simulink model "scenario1_TAC_5robots_plus"  (R2020b)
settings: Solver=FixedStepAuto  StartTime=0.0  StopTime=40.0  FixedStep=1e-2  RelTol=1e-3
libraries: simulink x6
(part 1 of 2)
settings Model: Creator=Admin  LastModifiedBy=Admin

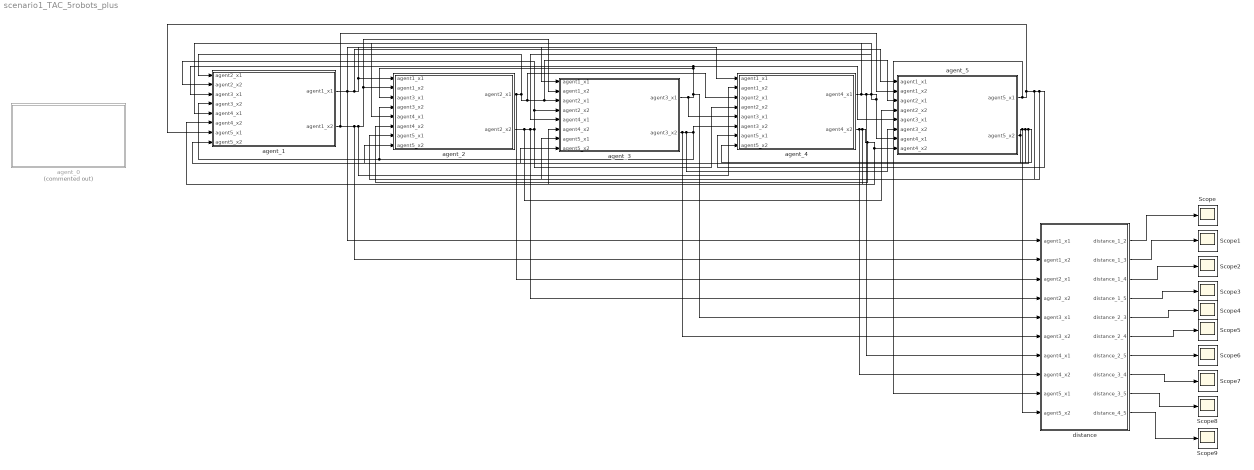
== system scenario1_TAC_5robots_plus ==
  Scope{,1..9} (10 alike) : Scope
  agent_0 : Subsystem  Commented=on
  agent_1 : Subsystem
  agent_2 : Subsystem
  agent_3 : Subsystem
  agent_4 : Subsystem
  agent_5 : Subsystem
  distance : MATLAB Function  TreatAsAtomicUnit=on
  wires:
  agent_2/1(agent2_x1) -> distance/3(agent2_x1), agent_1/1(agent2_x1), agent_4/3(agent2_x1), agent_5/3(agent2_x1), agent_3/3(agent2_x1)
  agent_1/1(agent1_x1) -> agent_4/1(agent1_x1), distance/1(agent1_x1), agent_5/1(agent1_x1), agent_3/1(agent1_x1), agent_2/1(agent1_x1)
  agent_1/2(agent1_x2) -> agent_5/2(agent1_x2), distance/2(agent1_x2), agent_4/2(agent1_x2), agent_3/2(agent1_x2), agent_2/2(agent1_x2)
  agent_2/2(agent2_x2) -> agent_5/4(agent2_x2), distance/4(agent2_x2), agent_4/4(agent2_x2), agent_1/2(agent2_x2), agent_3/4(agent2_x2)
  distance/1(distance_1_2) -> Scope/1
  agent_3/1(agent3_x1) -> agent_4/5(agent3_x1), distance/5(agent3_x1), agent_5/5(agent3_x1), agent_1/3(agent3_x1), agent_2/3(agent3_x1)
  agent_3/2(agent3_x2) -> distance/6(agent3_x2), agent_5/6(agent3_x2), agent_1/4(agent3_x2), agent_2/4(agent3_x2), agent_4/6(agent3_x2)
  agent_5/1(agent5_x1) -> distance/9(agent5_x1), agent_1/7(agent5_x1), agent_2/7(agent5_x1), agent_3/7(agent5_x1), agent_4/7(agent5_x1)
  agent_5/2(agent5_x2) -> distance/10(agent5_x2), agent_2/8(agent5_x2), agent_3/8(agent5_x2), agent_4/8(agent5_x2), agent_1/8(agent5_x2)
  agent_4/1(agent4_x1) -> agent_2/5(agent4_x1), agent_1/5(agent4_x1), agent_3/5(agent4_x1), agent_5/7(agent4_x1), distance/7(agent4_x1)
  agent_4/2(agent4_x2) -> distance/8(agent4_x2), agent_3/6(agent4_x2), agent_2/6(agent4_x2), agent_1/6(agent4_x2), agent_5/8(agent4_x2)
  distance/2(distance_1_3) -> Scope1/1
  distance/3(distance_1_4) -> Scope2/1
  distance/4(distance_1_5) -> Scope3/1
  distance/5(distance_2_3) -> Scope4/1
  distance/6(distance_2_4) -> Scope5/1
  distance/7(distance_2_5) -> Scope6/1
  distance/8(distance_3_4) -> Scope7/1
  distance/9(distance_3_5) -> Scope8/1
  distance/10(distance_4_5) -> Scope9/1

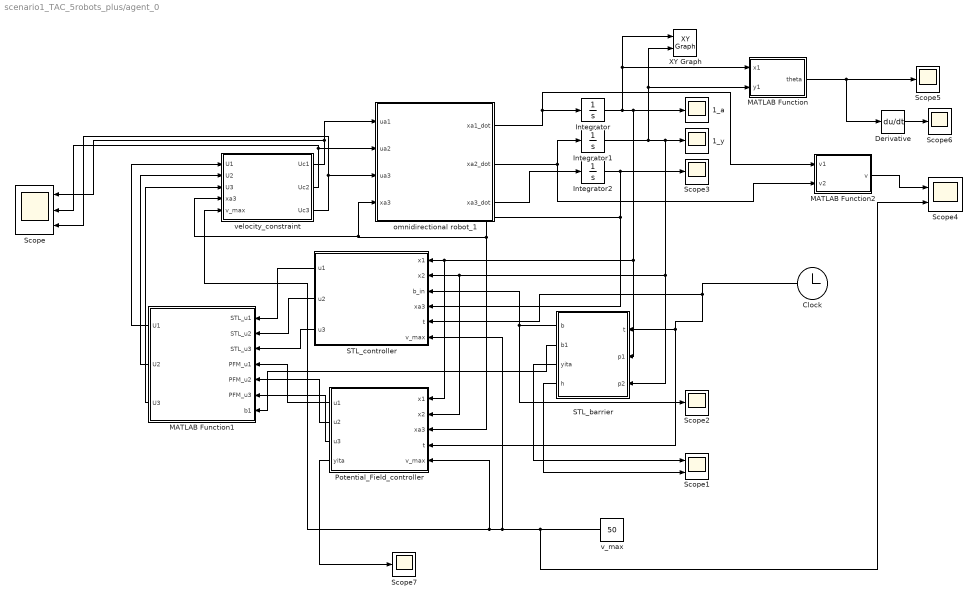
== system scenario1_TAC_5robots_plus/agent_0 ==
  1_a : Scope
  1_y : Scope
  Clock : Clock
  Derivative : Derivative
  Integrator : Integrator  InitialCondition=100
  Integrator1 : Integrator
  Integrator2 : Integrator
  MATLAB Function : MATLAB Function  TreatAsAtomicUnit=on
  MATLAB Function1 : MATLAB Function  TreatAsAtomicUnit=on
  MATLAB Function2 : MATLAB Function  TreatAsAtomicUnit=on
  Potential_Field_controller : MATLAB Function  TreatAsAtomicUnit=on
  "STL_barrier " : MATLAB Function  TreatAsAtomicUnit=on
  STL_controller : MATLAB Function  TreatAsAtomicUnit=on
  Scope : Scope  NumInputPorts=3
  Scope1 : Scope  NumInputPorts=2
  Scope{2..3,5..7} (5 alike) : Scope
  Scope4 : Scope  NumInputPorts=2
  XY Graph : simulink/Sinks/XY Graph  xmin=-15  xmax=100  ymin=-15  ymax=100  st=0.01
  omnidirectional robot_1 : MATLAB Function  TreatAsAtomicUnit=on
  v_max : Constant  Value=50
  velocity_constraint : MATLAB Function  TreatAsAtomicUnit=on
  wires:
  Potential_Field_controller/2(u2) -> MATLAB Function1/5(PFM_u2)
  velocity_constraint/2(Uc2) -> omnidirectional robot_1/2(ua2), Scope/2
  v_max/1 -> Scope4/2, STL_controller/6(v_max), velocity_constraint/5(v_max), Potential_Field_controller/5(v_max)
  STL_controller/1(u1) -> MATLAB Function1/1(STL_u1)
  Integrator/1 -> MATLAB Function/1(x1), XY Graph/1, "STL_barrier "/2(p1), Potential_Field_controller/1(x1), STL_controller/1(x1), 1_a/1
  Clock/1 -> Potential_Field_controller/4(t), "STL_barrier "/1(t), STL_controller/5(t)
  MATLAB Function1/3(U3) -> velocity_constraint/3(U3)
  omnidirectional robot_1/2(xa2_dot) -> Integrator1/1, MATLAB Function2/2(v2)
  velocity_constraint/1(Uc1) -> Scope/1, omnidirectional robot_1/1(ua1)
  velocity_constraint/3(Uc3) -> Scope/3, omnidirectional robot_1/3(ua3)
  Integrator1/1 -> MATLAB Function/2(y1), XY Graph/2, "STL_barrier "/3(p2), Potential_Field_controller/2(x2), STL_controller/2(x2), 1_y/1
  MATLAB Function/1(theta) -> Derivative/1, Scope5/1
  omnidirectional robot_1/1(xa1_dot) -> MATLAB Function2/1(v1), Integrator/1
  omnidirectional robot_1/3(xa3_dot) -> Integrator2/1
  "STL_barrier "/3(yita) -> Scope1/1
  STL_controller/3(u3) -> MATLAB Function1/3(STL_u3)
  Integrator2/1 -> Potential_Field_controller/3(xa3), velocity_constraint/4(xa3), omnidirectional robot_1/4(xa3), STL_controller/4(xa3), Scope3/1
  Potential_Field_controller/1(u1) -> MATLAB Function1/4(PFM_u1)
  MATLAB Function1/1(U1) -> velocity_constraint/1(U1)
  Potential_Field_controller/4(yita) -> Scope7/1
  STL_controller/2(u2) -> MATLAB Function1/2(STL_u2)
  MATLAB Function2/1(v) -> Scope4/1
  "STL_barrier "/2(b1) -> MATLAB Function1/7(b1)
  Derivative/1 -> Scope6/1
  MATLAB Function1/2(U2) -> velocity_constraint/2(U2)
  "STL_barrier "/1(b) -> STL_controller/3(b_in), Scope2/1
  Potential_Field_controller/3(u3) -> MATLAB Function1/6(PFM_u3)
  "STL_barrier "/4(h) -> Scope1/2

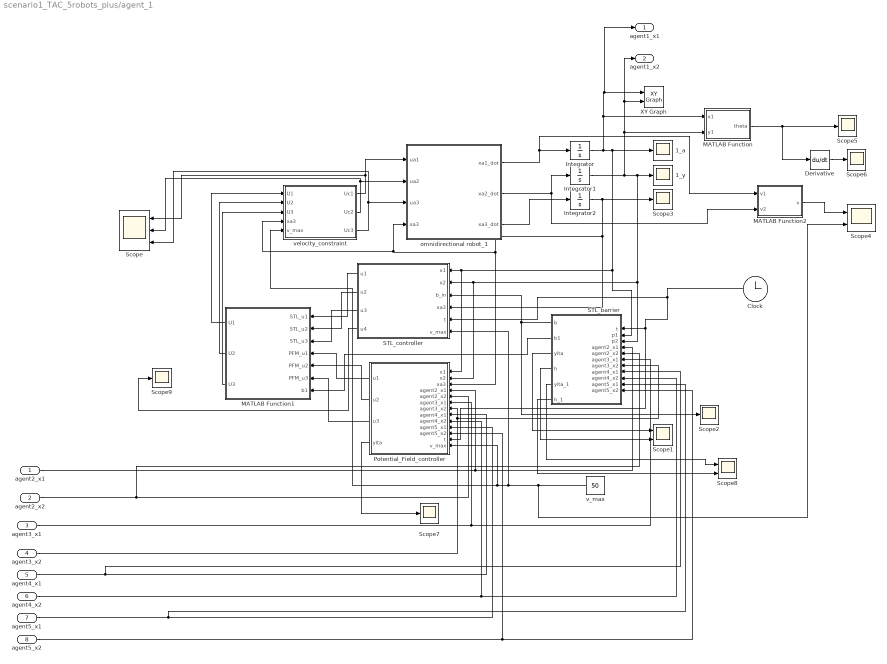
== system scenario1_TAC_5robots_plus/agent_1 ==
  agent2_x1 : Inport
  agent2_x2 : Inport  Port=2
  agent3_x1 : Inport  Port=3
  agent3_x2 : Inport  Port=4
  agent4_x1 : Inport  Port=5
  agent4_x2 : Inport  Port=6
  agent5_x1 : Inport  Port=7
  agent5_x2 : Inport  Port=8
  1_a : Scope
  1_y : Scope
  Clock : Clock
  Derivative : Derivative
  Integrator : Integrator  InitialCondition=0.5
  Integrator1 : Integrator
  Integrator2 : Integrator
  MATLAB Function : MATLAB Function  TreatAsAtomicUnit=on
  MATLAB Function1 : MATLAB Function  TreatAsAtomicUnit=on
  MATLAB Function2 : MATLAB Function  TreatAsAtomicUnit=on
  Potential_Field_controller : MATLAB Function  TreatAsAtomicUnit=on
  "STL_barrier " : MATLAB Function  TreatAsAtomicUnit=on
  STL_controller : MATLAB Function  TreatAsAtomicUnit=on
  Scope : Scope  NumInputPorts=3
  Scope1 : Scope  NumInputPorts=2
  Scope{2..3,5..7,9} (6 alike) : Scope
  Scope4 : Scope  NumInputPorts=2
  Scope8 : Scope  NumInputPorts=2
  XY Graph : simulink/Sinks/XY Graph  xmin=-15  xmax=100  ymin=-15  ymax=100  st=0.01
  omnidirectional robot_1 : MATLAB Function  TreatAsAtomicUnit=on
  v_max : Constant  Value=50
  velocity_constraint : MATLAB Function  TreatAsAtomicUnit=on
  agent1_x1 : Outport
  agent1_x2 : Outport  Port=2
  wires:
  Potential_Field_controller/2(u2) -> MATLAB Function1/5(PFM_u2)
  velocity_constraint/2(Uc2) -> omnidirectional robot_1/2(ua2), Scope/2
  v_max/1 -> Scope4/2, STL_controller/6(v_max), velocity_constraint/5(v_max), Potential_Field_controller/13(v_max)
  STL_controller/1(u1) -> MATLAB Function1/1(STL_u1)
  Integrator/1 -> MATLAB Function/1(x1), agent1_x1/1, XY Graph/1, "STL_barrier "/2(p1), Potential_Field_controller/1(x1), STL_controller/1(x1), 1_a/1
  Clock/1 -> Potential_Field_controller/12(t), "STL_barrier "/1(t), STL_controller/5(t)
  MATLAB Function1/3(U3) -> velocity_constraint/3(U3)
  omnidirectional robot_1/2(xa2_dot) -> Integrator1/1, MATLAB Function2/2(v2)
  velocity_constraint/1(Uc1) -> Scope/1, omnidirectional robot_1/1(ua1)
  velocity_constraint/3(Uc3) -> Scope/3, omnidirectional robot_1/3(ua3)
  Integrator1/1 -> MATLAB Function/2(y1), agent1_x2/1, XY Graph/2, "STL_barrier "/3(p2), Potential_Field_controller/2(x2), STL_controller/2(x2), 1_y/1
  MATLAB Function/1(theta) -> Derivative/1, Scope5/1
  omnidirectional robot_1/1(xa1_dot) -> MATLAB Function2/1(v1), Integrator/1
  omnidirectional robot_1/3(xa3_dot) -> Integrator2/1
  "STL_barrier "/3(yita) -> Scope1/1
  STL_controller/3(u3) -> MATLAB Function1/3(STL_u3)
  Integrator2/1 -> Potential_Field_controller/3(xa3), velocity_constraint/4(xa3), omnidirectional robot_1/4(xa3), STL_controller/4(xa3), Scope3/1
  Potential_Field_controller/1(u1) -> MATLAB Function1/4(PFM_u1)
  MATLAB Function1/1(U1) -> velocity_constraint/1(U1)
  Potential_Field_controller/4(yita) -> Scope7/1
  STL_controller/2(u2) -> MATLAB Function1/2(STL_u2)
  MATLAB Function2/1(v) -> Scope4/1
  "STL_barrier "/2(b1) -> MATLAB Function1/7(b1)
  Derivative/1 -> Scope6/1
  MATLAB Function1/2(U2) -> velocity_constraint/2(U2)
  "STL_barrier "/1(b) -> Scope2/1, STL_controller/3(b_in)
  Potential_Field_controller/3(u3) -> MATLAB Function1/6(PFM_u3)
  "STL_barrier "/4(h) -> Scope1/2
  agent2_x1/1 -> "STL_barrier "/4(agent2_x1), Potential_Field_controller/4(agent2_x1)
  agent2_x2/1 -> "STL_barrier "/5(agent2_x2), Potential_Field_controller/5(agent2_x2)
  agent3_x2/1 -> Potential_Field_controller/7(agent3_x2), "STL_barrier "/7(agent3_x2)
  agent4_x1/1 -> "STL_barrier "/8(agent4_x1), Potential_Field_controller/8(agent4_x1)
  agent4_x2/1 -> "STL_barrier "/9(agent4_x2), Potential_Field_controller/9(agent4_x2)
  agent5_x1/1 -> "STL_barrier "/10(agent5_x1), Potential_Field_controller/10(agent5_x1)
  agent5_x2/1 -> "STL_barrier "/11(agent5_x2), Potential_Field_controller/11(agent5_x2)
  agent3_x1/1 -> "STL_barrier "/6(agent3_x1), Potential_Field_controller/6(agent3_x1)
  "STL_barrier "/5(yita_1) -> Scope8/1
  "STL_barrier "/6(h_1) -> Scope8/2
  STL_controller/4(u4) -> Scope9/1

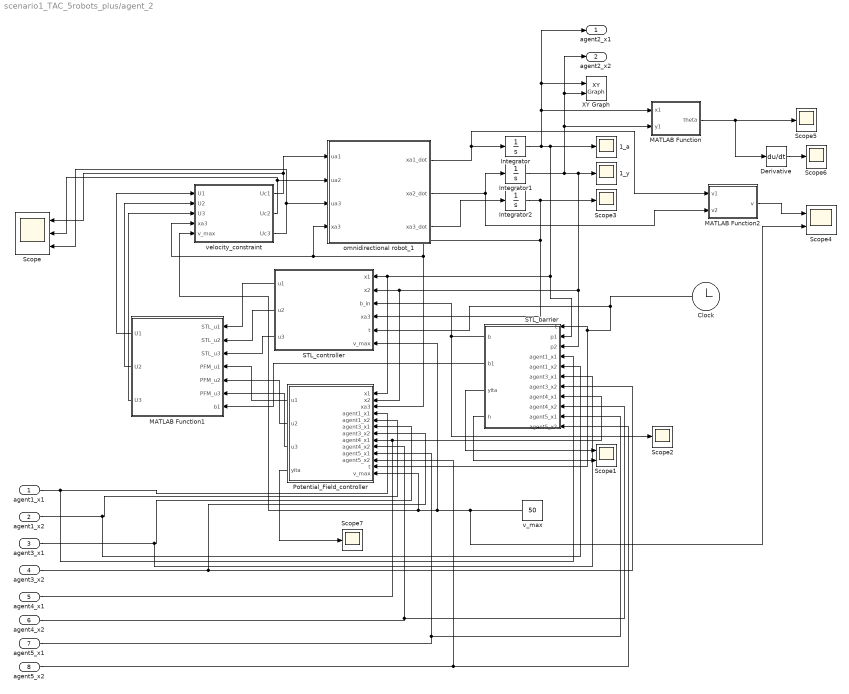
== system scenario1_TAC_5robots_plus/agent_2 ==
  agent1_x1 : Inport
  agent1_x2 : Inport  Port=2
  agent3_x1 : Inport  Port=3
  agent3_x2 : Inport  Port=4
  agent4_x1 : Inport  Port=5
  agent4_x2 : Inport  Port=6
  agent5_x1 : Inport  Port=7
  agent5_x2 : Inport  Port=8
  1_a : Scope
  1_y : Scope
  Clock : Clock
  Derivative : Derivative
  Integrator : Integrator  InitialCondition=99.5
  Integrator1 : Integrator
  Integrator2 : Integrator
  MATLAB Function : MATLAB Function  TreatAsAtomicUnit=on
  MATLAB Function1 : MATLAB Function  TreatAsAtomicUnit=on
  MATLAB Function2 : MATLAB Function  TreatAsAtomicUnit=on
  Potential_Field_controller : MATLAB Function  TreatAsAtomicUnit=on
  "STL_barrier " : MATLAB Function  TreatAsAtomicUnit=on
  STL_controller : MATLAB Function  TreatAsAtomicUnit=on
  Scope : Scope  NumInputPorts=3
  Scope1 : Scope  NumInputPorts=2
  Scope{2..3,5..7} (5 alike) : Scope
  Scope4 : Scope  NumInputPorts=2
  XY Graph : simulink/Sinks/XY Graph  xmin=-15  xmax=100  ymin=-15  ymax=100  st=0.01
  omnidirectional robot_1 : MATLAB Function  TreatAsAtomicUnit=on
  v_max : Constant  Value=50
  velocity_constraint : MATLAB Function  TreatAsAtomicUnit=on
  agent2_x1 : Outport
  agent2_x2 : Outport  Port=2
  wires:
  Potential_Field_controller/2(u2) -> MATLAB Function1/5(PFM_u2)
  velocity_constraint/2(Uc2) -> omnidirectional robot_1/2(ua2), Scope/2
  v_max/1 -> Scope4/2, STL_controller/6(v_max), velocity_constraint/5(v_max), Potential_Field_controller/13(v_max)
  STL_controller/1(u1) -> MATLAB Function1/1(STL_u1)
  Integrator/1 -> MATLAB Function/1(x1), agent2_x1/1, XY Graph/1, "STL_barrier "/2(p1), Potential_Field_controller/1(x1), STL_controller/1(x1), 1_a/1
  Clock/1 -> Potential_Field_controller/12(t), "STL_barrier "/1(t), STL_controller/5(t)
  MATLAB Function1/3(U3) -> velocity_constraint/3(U3)
  omnidirectional robot_1/2(xa2_dot) -> Integrator1/1, MATLAB Function2/2(v2)
  velocity_constraint/1(Uc1) -> Scope/1, omnidirectional robot_1/1(ua1)
  velocity_constraint/3(Uc3) -> Scope/3, omnidirectional robot_1/3(ua3)
  Integrator1/1 -> MATLAB Function/2(y1), agent2_x2/1, XY Graph/2, "STL_barrier "/3(p2), Potential_Field_controller/2(x2), STL_controller/2(x2), 1_y/1
  MATLAB Function/1(theta) -> Derivative/1, Scope5/1
  omnidirectional robot_1/1(xa1_dot) -> MATLAB Function2/1(v1), Integrator/1
  omnidirectional robot_1/3(xa3_dot) -> Integrator2/1
  "STL_barrier "/3(yita) -> Scope1/1
  STL_controller/3(u3) -> MATLAB Function1/3(STL_u3)
  Integrator2/1 -> Potential_Field_controller/3(xa3), velocity_constraint/4(xa3), omnidirectional robot_1/4(xa3), STL_controller/4(xa3), Scope3/1
  Potential_Field_controller/1(u1) -> MATLAB Function1/4(PFM_u1)
  MATLAB Function1/1(U1) -> velocity_constraint/1(U1)
  Potential_Field_controller/4(yita) -> Scope7/1
  STL_controller/2(u2) -> MATLAB Function1/2(STL_u2)
  MATLAB Function2/1(v) -> Scope4/1
  "STL_barrier "/2(b1) -> MATLAB Function1/7(b1)
  Derivative/1 -> Scope6/1
  MATLAB Function1/2(U2) -> velocity_constraint/2(U2)
  "STL_barrier "/1(b) -> STL_controller/3(b_in), Scope2/1
  Potential_Field_controller/3(u3) -> MATLAB Function1/6(PFM_u3)
  "STL_barrier "/4(h) -> Scope1/2
  agent1_x1/1 -> "STL_barrier "/4(agent1_x1), Potential_Field_controller/4(agent1_x1)
  agent1_x2/1 -> "STL_barrier "/5(agent1_x2), Potential_Field_controller/5(agent1_x2)
  agent3_x1/1 -> "STL_barrier "/6(agent3_x1), Potential_Field_controller/6(agent3_x1)
  agent3_x2/1 -> "STL_barrier "/7(agent3_x2), Potential_Field_controller/7(agent3_x2)
  agent4_x1/1 -> "STL_barrier "/8(agent4_x1), Potential_Field_controller/8(agent4_x1)
  agent4_x2/1 -> "STL_barrier "/9(agent4_x2), Potential_Field_controller/9(agent4_x2)
  agent5_x1/1 -> "STL_barrier "/10(agent5_x1), Potential_Field_controller/10(agent5_x1)
  agent5_x2/1 -> "STL_barrier "/11(agent5_x2), Potential_Field_controller/11(agent5_x2)

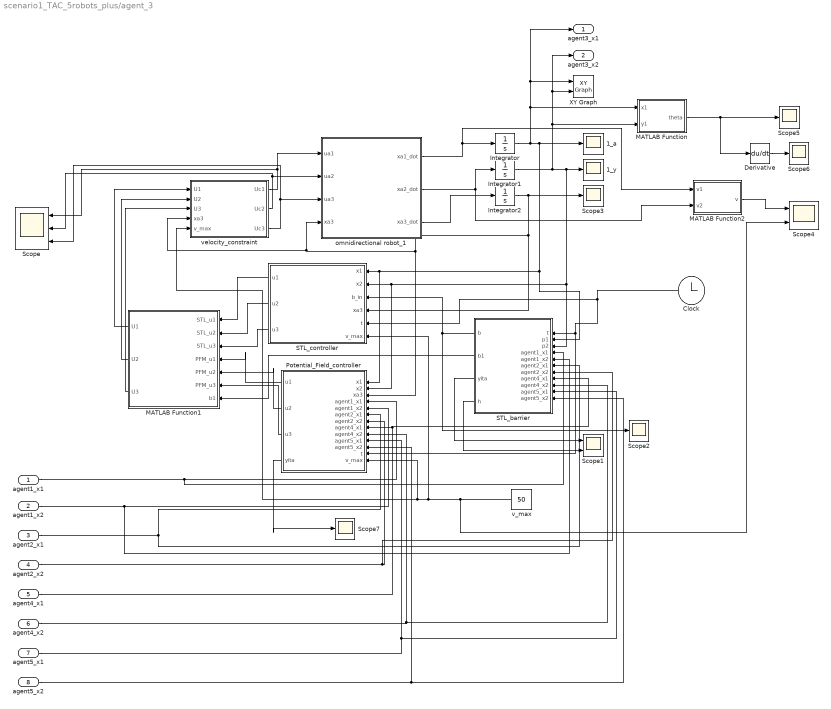
== system scenario1_TAC_5robots_plus/agent_3 ==
  agent1_x1 : Inport
  agent1_x2 : Inport  Port=2
  agent2_x1 : Inport  Port=3
  agent2_x2 : Inport  Port=4
  agent4_x1 : Inport  Port=5
  agent4_x2 : Inport  Port=6
  agent5_x1 : Inport  Port=7
  agent5_x2 : Inport  Port=8
  1_a : Scope
  1_y : Scope
  Clock : Clock
  Derivative : Derivative
  Integrator : Integrator  InitialCondition=50
  Integrator1 : Integrator  InitialCondition=100
  Integrator2 : Integrator
  MATLAB Function : MATLAB Function  TreatAsAtomicUnit=on
  MATLAB Function1 : MATLAB Function  TreatAsAtomicUnit=on
  MATLAB Function2 : MATLAB Function  TreatAsAtomicUnit=on
  Potential_Field_controller : MATLAB Function  TreatAsAtomicUnit=on
  "STL_barrier " : MATLAB Function  TreatAsAtomicUnit=on
  STL_controller : MATLAB Function  TreatAsAtomicUnit=on
  Scope : Scope  NumInputPorts=3
  Scope1 : Scope  NumInputPorts=2
  Scope{2..3,5..7} (5 alike) : Scope
  Scope4 : Scope  NumInputPorts=2
  XY Graph : simulink/Sinks/XY Graph  xmin=-15  xmax=100  ymin=-15  ymax=100  st=0.01
  omnidirectional robot_1 : MATLAB Function  TreatAsAtomicUnit=on
  v_max : Constant  Value=50
  velocity_constraint : MATLAB Function  TreatAsAtomicUnit=on
  agent3_x1 : Outport
  agent3_x2 : Outport  Port=2
  wires:
  Potential_Field_controller/2(u2) -> MATLAB Function1/5(PFM_u2)
  velocity_constraint/2(Uc2) -> omnidirectional robot_1/2(ua2), Scope/2
  v_max/1 -> Scope4/2, STL_controller/6(v_max), velocity_constraint/5(v_max), Potential_Field_controller/13(v_max)
  STL_controller/1(u1) -> MATLAB Function1/1(STL_u1)
  Integrator/1 -> MATLAB Function/1(x1), agent3_x1/1, XY Graph/1, "STL_barrier "/2(p1), Potential_Field_controller/1(x1), STL_controller/1(x1), 1_a/1
  Clock/1 -> Potential_Field_controller/12(t), "STL_barrier "/1(t), STL_controller/5(t)
  MATLAB Function1/3(U3) -> velocity_constraint/3(U3)
  omnidirectional robot_1/2(xa2_dot) -> Integrator1/1, MATLAB Function2/2(v2)
  velocity_constraint/1(Uc1) -> Scope/1, omnidirectional robot_1/1(ua1)
  velocity_constraint/3(Uc3) -> Scope/3, omnidirectional robot_1/3(ua3)
  Integrator1/1 -> MATLAB Function/2(y1), agent3_x2/1, XY Graph/2, "STL_barrier "/3(p2), Potential_Field_controller/2(x2), STL_controller/2(x2), 1_y/1
  MATLAB Function/1(theta) -> Derivative/1, Scope5/1
  omnidirectional robot_1/1(xa1_dot) -> MATLAB Function2/1(v1), Integrator/1
  omnidirectional robot_1/3(xa3_dot) -> Integrator2/1
  "STL_barrier "/3(yita) -> Scope1/1
  STL_controller/3(u3) -> MATLAB Function1/3(STL_u3)
  Integrator2/1 -> Potential_Field_controller/3(xa3), velocity_constraint/4(xa3), omnidirectional robot_1/4(xa3), STL_controller/4(xa3), Scope3/1
  Potential_Field_controller/1(u1) -> MATLAB Function1/4(PFM_u1)
  MATLAB Function1/1(U1) -> velocity_constraint/1(U1)
  Potential_Field_controller/4(yita) -> Scope7/1
  STL_controller/2(u2) -> MATLAB Function1/2(STL_u2)
  MATLAB Function2/1(v) -> Scope4/1
  "STL_barrier "/2(b1) -> MATLAB Function1/7(b1)
  Derivative/1 -> Scope6/1
  MATLAB Function1/2(U2) -> velocity_constraint/2(U2)
  "STL_barrier "/1(b) -> STL_controller/3(b_in), Scope2/1
  Potential_Field_controller/3(u3) -> MATLAB Function1/6(PFM_u3)
  "STL_barrier "/4(h) -> Scope1/2
  agent1_x1/1 -> "STL_barrier "/4(agent1_x1), Potential_Field_controller/4(agent1_x1)
  agent1_x2/1 -> "STL_barrier "/5(agent1_x2), Potential_Field_controller/5(agent1_x2)
  agent2_x1/1 -> Potential_Field_controller/6(agent2_x1), "STL_barrier "/6(agent2_x1)
  agent2_x2/1 -> "STL_barrier "/7(agent2_x2), Potential_Field_controller/7(agent2_x2)
  agent4_x1/1 -> "STL_barrier "/8(agent4_x1), Potential_Field_controller/8(agent4_x1)
  agent4_x2/1 -> "STL_barrier "/9(agent4_x2), Potential_Field_controller/9(agent4_x2)
  agent5_x1/1 -> "STL_barrier "/10(agent5_x1), Potential_Field_controller/10(agent5_x1)
  agent5_x2/1 -> "STL_barrier "/11(agent5_x2), Potential_Field_controller/11(agent5_x2)

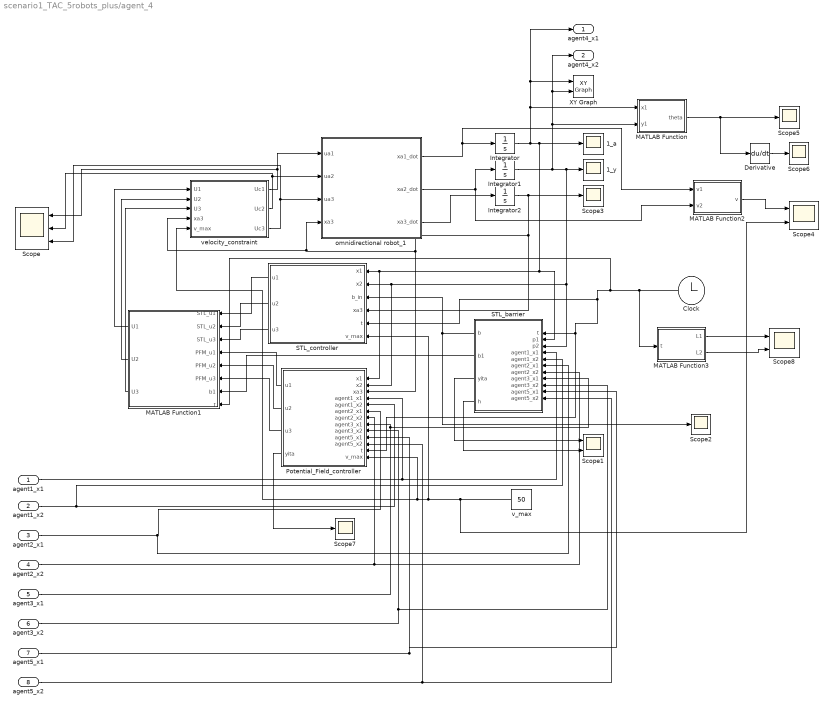
== system scenario1_TAC_5robots_plus/agent_4 ==
  agent1_x1 : Inport
  agent1_x2 : Inport  Port=2
  agent2_x1 : Inport  Port=3
  agent2_x2 : Inport  Port=4
  agent3_x1 : Inport  Port=5
  agent3_x2 : Inport  Port=6
  agent5_x1 : Inport  Port=7
  agent5_x2 : Inport  Port=8
  1_a : Scope
  1_y : Scope
  Clock : Clock
  Derivative : Derivative
  Integrator : Integrator
  Integrator1 : Integrator  InitialCondition=50
  Integrator2 : Integrator
  MATLAB Function : MATLAB Function  TreatAsAtomicUnit=on
  MATLAB Function1 : MATLAB Function  TreatAsAtomicUnit=on
  MATLAB Function2 : MATLAB Function  TreatAsAtomicUnit=on
  MATLAB Function3 : MATLAB Function  TreatAsAtomicUnit=on
  Potential_Field_controller : MATLAB Function  TreatAsAtomicUnit=on
  "STL_barrier " : MATLAB Function  TreatAsAtomicUnit=on
  STL_controller : MATLAB Function  TreatAsAtomicUnit=on
  Scope : Scope  NumInputPorts=3
  Scope1 : Scope  NumInputPorts=2
  Scope{2..3,5..7} (5 alike) : Scope
  Scope4 : Scope  NumInputPorts=2
  Scope8 : Scope  NumInputPorts=2
  XY Graph : simulink/Sinks/XY Graph  xmin=-15  xmax=100  ymin=-15  ymax=100  st=0.01
  omnidirectional robot_1 : MATLAB Function  TreatAsAtomicUnit=on
  v_max : Constant  Value=50
  velocity_constraint : MATLAB Function  TreatAsAtomicUnit=on
  agent4_x1 : Outport
  agent4_x2 : Outport  Port=2
  wires:
  Potential_Field_controller/2(u2) -> MATLAB Function1/5(PFM_u2)
  velocity_constraint/2(Uc2) -> omnidirectional robot_1/2(ua2), Scope/2
  v_max/1 -> Scope4/2, STL_controller/6(v_max), velocity_constraint/5(v_max), Potential_Field_controller/13(v_max)
  STL_controller/1(u1) -> MATLAB Function1/1(STL_u1)
  Integrator/1 -> MATLAB Function/1(x1), agent4_x1/1, XY Graph/1, "STL_barrier "/2(p1), Potential_Field_controller/1(x1), STL_controller/1(x1), 1_a/1
  Clock/1 -> MATLAB Function3/1(t), MATLAB Function1/8(t), Potential_Field_controller/12(t), "STL_barrier "/1(t), STL_controller/5(t)
  MATLAB Function1/3(U3) -> velocity_constraint/3(U3)
  omnidirectional robot_1/2(xa2_dot) -> Integrator1/1, MATLAB Function2/2(v2)
  velocity_constraint/1(Uc1) -> Scope/1, omnidirectional robot_1/1(ua1)
  velocity_constraint/3(Uc3) -> Scope/3, omnidirectional robot_1/3(ua3)
  Integrator1/1 -> MATLAB Function/2(y1), agent4_x2/1, XY Graph/2, "STL_barrier "/3(p2), Potential_Field_controller/2(x2), STL_controller/2(x2), 1_y/1
  MATLAB Function/1(theta) -> Derivative/1, Scope5/1
  omnidirectional robot_1/1(xa1_dot) -> MATLAB Function2/1(v1), Integrator/1
  omnidirectional robot_1/3(xa3_dot) -> Integrator2/1
  "STL_barrier "/3(yita) -> Scope1/1
  STL_controller/3(u3) -> MATLAB Function1/3(STL_u3)
  Integrator2/1 -> Potential_Field_controller/3(xa3), velocity_constraint/4(xa3), omnidirectional robot_1/4(xa3), STL_controller/4(xa3), Scope3/1
  Potential_Field_controller/1(u1) -> MATLAB Function1/4(PFM_u1)
  MATLAB Function1/1(U1) -> velocity_constraint/1(U1)
  Potential_Field_controller/4(yita) -> Scope7/1
  STL_controller/2(u2) -> MATLAB Function1/2(STL_u2)
  MATLAB Function2/1(v) -> Scope4/1
  "STL_barrier "/2(b1) -> MATLAB Function1/7(b1)
  Derivative/1 -> Scope6/1
  MATLAB Function1/2(U2) -> velocity_constraint/2(U2)
  "STL_barrier "/1(b) -> STL_controller/3(b_in), Scope2/1
  Potential_Field_controller/3(u3) -> MATLAB Function1/6(PFM_u3)
  "STL_barrier "/4(h) -> Scope1/2
  agent1_x1/1 -> "STL_barrier "/4(agent1_x1), Potential_Field_controller/4(agent1_x1)
  agent1_x2/1 -> "STL_barrier "/5(agent1_x2), Potential_Field_controller/5(agent1_x2)
  agent2_x1/1 -> "STL_barrier "/6(agent2_x1), Potential_Field_controller/6(agent2_x1)
  agent2_x2/1 -> "STL_barrier "/7(agent2_x2), Potential_Field_controller/7(agent2_x2)
  agent3_x1/1 -> "STL_barrier "/8(agent3_x1), Potential_Field_controller/8(agent3_x1)
  agent3_x2/1 -> "STL_barrier "/9(agent3_x2), Potential_Field_controller/9(agent3_x2)
  agent5_x1/1 -> "STL_barrier "/10(agent5_x1), Potential_Field_controller/10(agent5_x1)
  agent5_x2/1 -> "STL_barrier "/11(agent5_x2), Potential_Field_controller/11(agent5_x2)
  MATLAB Function3/1(L1) -> Scope8/1
  MATLAB Function3/2(L2) -> Scope8/2

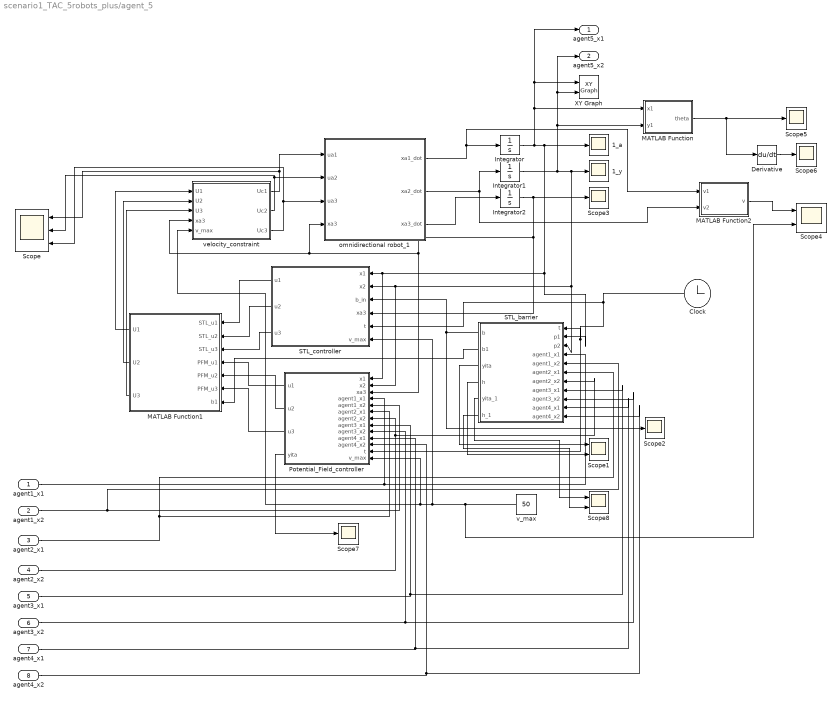
== system scenario1_TAC_5robots_plus/agent_5 ==
  agent1_x1 : Inport
  agent1_x2 : Inport  Port=2
  agent2_x1 : Inport  Port=3
  agent2_x2 : Inport  Port=4
  agent3_x1 : Inport  Port=5
  agent3_x2 : Inport  Port=6
  agent4_x1 : Inport  Port=7
  agent4_x2 : Inport  Port=8
  1_a : Scope
  1_y : Scope
  Clock : Clock
  Derivative : Derivative
  Integrator : Integrator
  Integrator1 : Integrator  InitialCondition=100
  Integrator2 : Integrator
  MATLAB Function : MATLAB Function  TreatAsAtomicUnit=on
  MATLAB Function1 : MATLAB Function  TreatAsAtomicUnit=on
  MATLAB Function2 : MATLAB Function  TreatAsAtomicUnit=on
  Potential_Field_controller : MATLAB Function  TreatAsAtomicUnit=on
  "STL_barrier " : MATLAB Function  TreatAsAtomicUnit=on
  STL_controller : MATLAB Function  TreatAsAtomicUnit=on
  Scope : Scope  NumInputPorts=3
  Scope1 : Scope  NumInputPorts=2
  Scope{2..3,5..7} (5 alike) : Scope
  Scope4 : Scope  NumInputPorts=2
  Scope8 : Scope  NumInputPorts=2
  XY Graph : simulink/Sinks/XY Graph  xmin=-15  xmax=100  ymin=-15  ymax=100  st=0.01
  omnidirectional robot_1 : MATLAB Function  TreatAsAtomicUnit=on
  v_max : Constant  Value=50
  velocity_constraint : MATLAB Function  TreatAsAtomicUnit=on
  agent5_x1 : Outport
  agent5_x2 : Outport  Port=2
  wires:
  Potential_Field_controller/2(u2) -> MATLAB Function1/5(PFM_u2)
  velocity_constraint/2(Uc2) -> omnidirectional robot_1/2(ua2), Scope/2
  v_max/1 -> Scope4/2, STL_controller/6(v_max), velocity_constraint/5(v_max), Potential_Field_controller/13(v_max)
  STL_controller/1(u1) -> MATLAB Function1/1(STL_u1)
  Integrator/1 -> MATLAB Function/1(x1), agent5_x1/1, XY Graph/1, "STL_barrier "/2(p1), Potential_Field_controller/1(x1), STL_controller/1(x1), 1_a/1
  Clock/1 -> Potential_Field_controller/12(t), "STL_barrier "/1(t), STL_controller/5(t)
  MATLAB Function1/3(U3) -> velocity_constraint/3(U3)
  omnidirectional robot_1/2(xa2_dot) -> Integrator1/1, MATLAB Function2/2(v2)
  velocity_constraint/1(Uc1) -> Scope/1, omnidirectional robot_1/1(ua1)
  velocity_constraint/3(Uc3) -> Scope/3, omnidirectional robot_1/3(ua3)
  Integrator1/1 -> MATLAB Function/2(y1), agent5_x2/1, XY Graph/2, "STL_barrier "/3(p2), Potential_Field_controller/2(x2), STL_controller/2(x2), 1_y/1
  MATLAB Function/1(theta) -> Derivative/1, Scope5/1
  omnidirectional robot_1/1(xa1_dot) -> MATLAB Function2/1(v1), Integrator/1
  omnidirectional robot_1/3(xa3_dot) -> Integrator2/1
  "STL_barrier "/3(yita) -> Scope1/1
  STL_controller/3(u3) -> MATLAB Function1/3(STL_u3)
  Integrator2/1 -> Potential_Field_controller/3(xa3), velocity_constraint/4(xa3), omnidirectional robot_1/4(xa3), STL_controller/4(xa3), Scope3/1
  Potential_Field_controller/1(u1) -> MATLAB Function1/4(PFM_u1)
  MATLAB Function1/1(U1) -> velocity_constraint/1(U1)
  Potential_Field_controller/4(yita) -> Scope7/1
  STL_controller/2(u2) -> MATLAB Function1/2(STL_u2)
  MATLAB Function2/1(v) -> Scope4/1
  "STL_barrier "/2(b1) -> MATLAB Function1/7(b1)
  Derivative/1 -> Scope6/1
  MATLAB Function1/2(U2) -> velocity_constraint/2(U2)
  "STL_barrier "/1(b) -> Scope2/1, STL_controller/3(b_in)
  Potential_Field_controller/3(u3) -> MATLAB Function1/6(PFM_u3)
  "STL_barrier "/4(h) -> Scope1/2
  agent1_x1/1 -> "STL_barrier "/4(agent1_x1), Potential_Field_controller/4(agent1_x1)
  agent1_x2/1 -> "STL_barrier "/5(agent1_x2), Potential_Field_controller/5(agent1_x2)
  agent2_x1/1 -> "STL_barrier "/6(agent2_x1), Potential_Field_controller/6(agent2_x1)
  agent2_x2/1 -> "STL_barrier "/7(agent2_x2), Potential_Field_controller/7(agent2_x2)
  agent3_x1/1 -> "STL_barrier "/8(agent3_x1), Potential_Field_controller/8(agent3_x1)
  agent3_x2/1 -> "STL_barrier "/9(agent3_x2), Potential_Field_controller/9(agent3_x2)
  agent4_x1/1 -> "STL_barrier "/10(agent4_x1), Potential_Field_controller/10(agent4_x1)
  agent4_x2/1 -> "STL_barrier "/11(agent4_x2), Potential_Field_controller/11(agent4_x2)
  "STL_barrier "/5(yita_1) -> Scope8/1
  "STL_barrier "/6(h_1) -> Scope8/2

== matlab function scenario1_TAC_5robots_plus/agent_1/MATLAB Function1 ==
  data: STL_u1 input; U1 output; STL_u2 input; STL_u3 input; PFM_u1 input; PFM_u2 input; PFM_u3 input; b1 input; U2 output; U3 output
function [U1,U2,U3] = fcn(STL_u1,STL_u2,STL_u3,PFM_u1,PFM_u2,PFM_u3,b1)
U_goal=[STL_u1;STL_u2;STL_u3];
U_obs=[PFM_u1;PFM_u2;PFM_u3];
k=0.15;
lambda=1-exp(-k*max(b1,0));
U=lambda*U_goal+(1-lambda)*U_obs;
U1=0;U2=0;U3=0;
U1=U(1,1);
U2=U(2,1);
U3=U(3,1);

== matlab function scenario1_TAC_5robots_plus/agent_2/MATLAB Function ==
  data: x1 input; theta output; y1 input
function theta = fcn(x1, y1)
theta=atan2(y1,x1);

== matlab function scenario1_TAC_5robots_plus/agent_2/MATLAB Function1 ==
  data: STL_u1 input; U1 output; STL_u2 input; STL_u3 input; PFM_u1 input; PFM_u2 input; PFM_u3 input; b1 input; U2 output; U3 output
function [U1,U2,U3] = fcn(STL_u1,STL_u2,STL_u3,PFM_u1,PFM_u2,PFM_u3,b1)
U_goal=[STL_u1;STL_u2;STL_u3];
U_obs=[PFM_u1;PFM_u2;PFM_u3];
k=0.15;
lambda=1-exp(-k*max(b1,0));
U=lambda*U_goal+(1-lambda)*U_obs;
U1=0;U2=0;U3=0;
U1=U(1,1);
U2=U(2,1);
U3=U(3,1);

== matlab function scenario1_TAC_5robots_plus/agent_2/MATLAB Function2 ==
  data: v1 input; v output; v2 input
function v = fcn(v1, v2)
v=sqrt(v1^2+v2^2);

== matlab function scenario1_TAC_5robots_plus/agent_2/Potential_Field_controller ==
  data: x1 input; x2 input; u1 output; xa3 input; agent1_x1 input; agent1_x2 input; agent3_x1 input; agent3_x2 input; agent4_x1 input; agent4_x2 input; agent5_x1 input; agent5_x2 input; t input; u2 output; u3 output; v_max input; yita output
function [u1,u2,u3,yita] = fcn(x1, x2, xa3,agent1_x1,agent1_x2,agent3_x1,agent3_x2,agent4_x1,agent4_x2,agent5_x1,agent5_x2,t,v_max)
coder.extrinsic('Calculate_gradient');
coder.extrinsic('Calculate_gradient_V1');
coder.extrinsic('Calculate_gradient_V1_yita');
coder.extrinsic('Calculate_gradient_static_d_1');
coder.extrinsic('Calculate_gradient_static_d_2');
coder.extrinsic('Calculate_gradient_dynamic');
coder.extrinsic('compute_convex_hull');
coder.extrinsic('PVF_optimizer');
coder.extrinsic('add_random');
yita=0;

A1=[-1,0;0,-1];
if t<20
    F=[0,200];
elseif t>=20 && t<41
     F=[100,0];
else
    F=[200,0];
end
obs=[50,50];
Robs_s=20;
r_obs=16;
distance=sqrt((x1-90)^2+(x2-90)^2);
gradient_x=0;gradient_y=0;
Dgradient_x=0;Dgradient_y=0;
agent1_gradient_x=0;agent1_gradient_y=0;
agent3_gradient_x=0;agent3_gradient_y=0;
agent4_gradient_x=0;agent4_gradient_y=0;
agent5_gradient_x=0;agent5_gradient_y=0;
[gradient_x,gradient_y]=Calculate_gradient(x1,x2,A1,F,50,50,Robs_s);
[agent1_gradient_x,agent1_gradient_y]=Calculate_gradient_dynamic(x1,x2,A1,F,agent1_x1,agent1_x2,10);
[agent3_gradient_x,agent3_gradient_y]=Calculate_gradient_dynamic(x1,x2,A1,F,agent3_x1,agent3_x2,10);
[agent4_gradient_x,agent4_gradient_y]=Calculate_gradient_dynamic(x1,x2,A1,F,agent4_x1,agent4_x2,10);
[agent5_gradient_x,agent5_gradient_y]=Calculate_gradient_dynamic(x1,x2,A1,F,agent5_x1,agent5_x2,10);
if sqrt((x1-agent1_x1)^2+(x2-agent1_x2)^2)<=30 %agent2 and agent1
    gradient_x=gradient_x+agent1_gradient_x;
    gradient_y=gradient_y+agent1_gradient_y;  
end
if sqrt((x1-agent3_x1)^2+(x2-agent3_x2)^2)<=30 %agent2 and agent3
    gradient_x=gradient_x+agent3_gradient_x;
    gradient_y=gradient_y+agent3_gradient_y; 
end
if sqrt((x1-agent4_x1)^2+(x2-agent4_x2)^2)<=30 %agent2 and agent4
    gradient_x=gradient_x+agent4_gradient_x;
    gradient_y=gradient_y+agent4_gradient_y; 
end
if sqrt((x1-agent5_x1)^2+(x2-agent5_x2)^2)<=30 %agent2 and agent5
    gradient_x=gradient_x+agent5_gradient_x;
    gradient_y=gradient_y+agent5_gradient_y; 
end
gradient_x=gradient_x;
gradient_y=gradient_y; 
gradient_z=0;
Gradient_all=[gradient_x;gradient_y;gradient_z];



Li=0.2;
Bi=[0,cos(pi/6),-cos(pi/6);
    -1,sin(pi/6),sin(pi/6);
    Li,Li,Li;];

R1=[cos(xa3),-sin(xa3),0;
    sin(xa3),cos(xa3),0;
    0,0,1;];
R=0.02;

gx=R1*inv(Bi')*R;
A=Gradient_all'*gx;
% A=[A;-gx];
%H=[1];
%H=[1,0;0,1];
%H=[0,0,0;0,0,0;0,0,0];

 H1=[1,0,0;0,1,0;0,0,0];
 H=(1/2)*gx'*H1*gx;
b=[0];
% b=[0;5000;5000;5000];
Gain=50;
Gradient_final=Gain*Gradient_all;
F=[-2*gx'*H1'*Gradient_final];
%=[];
u1=0;u2=0;u3=0;
U=PVF_optimizer(H,b,A,F,distance,gradient_x,gradient_y);

u1=U(1,1);
u2=U(2,1);
u3=U(3,1);

== matlab function scenario1_TAC_5robots_plus/agent_2/STL_barrier  ==
  data: b output; b1 output; yita output; h output; t input; p1 input; p2 input; agent1_x1 input; agent1_x2 input; agent3_x1 input; agent3_x2 input; agent4_x1 input; agent4_x2 input; agent5_x1 input; agent5_x2 input
function [b,b1,yita,h] = fcn(t,p1,p2,agent1_x1,agent1_x2,agent3_x1,agent3_x2,agent4_x1,agent4_x2,agent5_x1,agent5_x2)
if t<20
    d1=0;
    d2=100;
elseif t>=20 && t<41
    d1=50;
    d2=0;
else
    d1=100;
    d2=0;  
end

obs1=50;
obs2=50;
if t<20
b=145*exp(-0.24*t)+5-sqrt( (p1-d1)^2 + (p2-d2)^2 );
yita=-145*exp(-0.24*t)+5;
h=10-sqrt( (p1-d1)^2 + (p2-d2)^2 );
elseif t>=20 && t<41
    b=110*exp(-0.276*(t-20))+5-sqrt( (p1-d1)^2 + (p2-d2)^2 );
   yita=-110*exp(-0.276*(t-20))+5;
    h=10-sqrt( (p1-d1)^2 + (p2-d2)^2 );
else
   b=145*exp(-0.24*(t-40))+5-sqrt( (p1-d1)^2 + (p2-d2)^2 );
   yita=-145*exp(-0.24*(t-40))+5;
   h=10-sqrt( (p1-d1)^2 + (p2-d2)^2 );
end
% b11=sqrt( (p1-x1_agent2)^2 + (p2-x2_agent2)^2 )-10 %collision avoidence with agent2
bobs=sqrt( (p1-obs1)^2 + (p2-obs2)^2 )-20;%collision avoidence with obstacle (50,50)
b21=sqrt( (p1-agent1_x1)^2 + (p2-agent1_x2)^2 )-10;%collision avoidence with agent1
b23=sqrt( (p1-agent3_x1)^2 + (p2-agent3_x2)^2 )-10;%collision avoidence with agent3
b24=sqrt( (p1-agent4_x1)^2 + (p2-agent4_x2)^2 )-10;%collision avoidence with agent4
b25=sqrt( (p1-agent5_x1)^2 + (p2-agent5_x2)^2 )-10;%collision avoidence with agent5
% b13=sqrt( (p1-centerjk_1)^2 + (p2-centerjk_2)^2 )-R_jk_s;%collision avoidence with nominal
% b14=sqrt( (p1-60)^2 + (p2-85)^2 )-18; %static dynamic obstacle
% b15=sqrt( (p1-20)^2 + (p2-80)^2 )-10; %static dynamic obstacle


b1=-(1/20)*log(exp(-20*bobs)+exp(-20*b21)+exp(-20*b23)+exp(-20*b24)+exp(-20*b25));

% b1=-(1/20)*log(exp(-20*b11)+exp(-20*b12)+exp(-20*b14)+exp(-20*b15));%+log(2);

== matlab function scenario1_TAC_5robots_plus/agent_2/STL_controller ==
  data: x1 input; x2 input; b_in input; u1 output; xa3 input; u2 output; u3 output; t input; v_max input
function [u1,u2,u3]= fcn(x1, x2, b_in, xa3,t, v_max)
coder.extrinsic('quadoptimizer');
%coder.extrinsic('save');
if t<20
    d1=0; d2=100;
elseif t>=20 && t<41
   d1=50; d2=0; 
else
   d1=100; d2=0; 
end

partial_b=(1/2)*((x1-d1)^2+(x2-d2)^2)^(-1/2);
partial_b_x=[-2*partial_b*(x1-d1),-2*partial_b*(x2-d2),0];


Li=0.2;
Bi=[0,cos(pi/6),-cos(pi/6);
    -1,sin(pi/6),sin(pi/6);
    Li,Li,Li;];

R1=[cos(xa3),-sin(xa3),0;
    sin(xa3),cos(xa3),0;
    0,0,1;];
R=0.02;
gx=R1*inv(Bi')*R;

A=partial_b_x*gx;
% A=[A;-gx];
H=[1,0,0;0,1,0;0,0,1];
%H=[1];
if t<20
    b=5*b_in-0.24*145*exp(-0.24*t)-10;
elseif t>=20 && t<41
    b=5*b_in-0.276*110*exp(-0.276*(t-20))-10;
else
    b=20*b_in-0.24*145*exp(-0.24*(t-40))-100;
end
% b=[b;5000;5000;5000];


u1=0;u2=0;u3=0;
U=[0;0;0];
U=quadoptimizer(H,b,A);

%U=quadprod(H,[],-A,b);
% V=[0;0;0];
% V=gx*U;
% if V(1,1)^2+V(2,1)^2<=v_max^2
%      U(1,1)= U(1,1);
%      U(2,1)= U(2,1);
% else 
%     U(1,1)=sqrt(v_max^2/(V(1,1)^2+V(2,1)^2))*U(1,1);
%     U(2,1)=sqrt(v_max^2/(V(1,1)^2+V(2,1)^2))*U(2,1);
% end


u1=U(1,1);
u2=U(2,1);
u3=U(3,1);

== matlab function scenario1_TAC_5robots_plus/agent_2/omnidirectional robot_1 ==
  data: ua1 input; xa1_dot output; ua2 input; ua3 input; xa3 input; xa2_dot output; xa3_dot output
function [xa1_dot,xa2_dot,xa3_dot]= fcn(ua1,ua2,ua3,xa3)

Li=0.2;
Bi=[0,cos(pi/6),-cos(pi/6);
    -1,sin(pi/6),sin(pi/6);
    Li,Li,Li;];

R1=[cos(xa3),-sin(xa3),0;
    sin(xa3),cos(xa3),0;
    0,0,1;];
R=0.02;
A=R1*inv(Bi')*R*[ua1;ua2;ua3];
xa1_dot=A(1,1);
xa2_dot=A(2,1);
xa3_dot=A(3,1);

== matlab function scenario1_TAC_5robots_plus/agent_2/velocity_constraint ==
  data: U1 input; Uc1 output; U2 input; U3 input; Uc2 output; Uc3 output; xa3 input; v_max input
function [Uc1,Uc2,Uc3] = fcn(U1,U2,U3,xa3,v_max)

Li=0.2;
Bi=[0,cos(pi/6),-cos(pi/6);
    -1,sin(pi/6),sin(pi/6);
    Li,Li,Li;];

R1=[cos(xa3),-sin(xa3),0;
    sin(xa3),cos(xa3),0;
    0,0,1;];
R=0.02;
gx=R1*inv(Bi')*R;

U=[U1;U2;U3];
V=[0;0;0];
V=gx*U;
if V(1,1)^2+V(2,1)^2<=v_max^2
     U(1,1)= U(1,1);
     U(2,1)= U(2,1);
else 
    U(1,1)=sqrt(v_max^2/(V(1,1)^2+V(2,1)^2))*U(1,1);
    U(2,1)=sqrt(v_max^2/(V(1,1)^2+V(2,1)^2))*U(2,1);
    U(3,1)=sqrt(v_max^2/(V(1,1)^2+V(2,1)^2))*U(3,1);
end

Uc1=U(1,1);
Uc2=U(2,1);
Uc3=U(3,1);

== matlab function scenario1_TAC_5robots_plus/agent_0/MATLAB Function ==
  data: x1 input; theta output; y1 input
function theta = fcn(x1, y1)
theta=atan2(y1,x1);

== matlab function scenario1_TAC_5robots_plus/agent_0/MATLAB Function1 ==
  data: STL_u1 input; U1 output; STL_u2 input; STL_u3 input; PFM_u1 input; PFM_u2 input; PFM_u3 input; b1 input; U2 output; U3 output
function [U1,U2,U3] = fcn(STL_u1,STL_u2,STL_u3,PFM_u1,PFM_u2,PFM_u3,b1)
U_goal=[STL_u1;STL_u2;STL_u3];
U_obs=[PFM_u1;PFM_u2;PFM_u3];
k=0.15;
lambda=1-exp(-k*max(b1,0));
U=lambda*U_goal+(1-lambda)*U_obs;
U1=0;U2=0;U3=0;
U1=U(1,1);
U2=U(2,1);
U3=U(3,1);

== matlab function scenario1_TAC_5robots_plus/agent_0/MATLAB Function2 ==
  data: v1 input; v output; v2 input
function v = fcn(v1, v2)
v=sqrt(v1^2+v2^2);

== matlab function scenario1_TAC_5robots_plus/agent_0/Potential_Field_controller ==
  data: x1 input; x2 input; u1 output; xa3 input; t input; u2 output; u3 output; v_max input; yita output
function [u1,u2,u3,yita] = fcn(x1, x2, xa3,t,v_max)
coder.extrinsic('Calculate_gradient');
coder.extrinsic('Calculate_gradient_V1');
coder.extrinsic('Calculate_gradient_V1_yita');
coder.extrinsic('Calculate_gradient_static_d_1');
coder.extrinsic('Calculate_gradient_static_d_2');
coder.extrinsic('compute_convex_hull');
coder.extrinsic('PVF_optimizer');
coder.extrinsic('add_random');
yita=0;

A1=[-1,0;0,-1];
if t<20
    F=[0,200];
elseif t>=20 && t<40
     F=[0,200];
else
    F=[200,0];
end
obs=[50,50];
Robs_s=20;
r_obs=16;
distance=sqrt((x1-90)^2+(x2-90)^2);
gradient_x=0;gradient_y=0;
Dgradient_x=0;Dgradient_y=0;
D1gradient_x=0;D1gradient_y=0;D2gradient_x=0;D2gradient_y=0;
[gradient_x,gradient_y]=Calculate_gradient(x1,x2,A1,F,50,50,Robs_s);
% [D1gradient_x,D1gradient_y]=Calculate_gradient_static_d_1(x1,x2,A1,F,60,85,15);
% [D2gradient_x,D2gradient_y]=Calculate_gradient_static_d_2(x1,x2,A1,F,20,80,10);
% if t<11
% gradient_x=gradient_x+D1gradient_x;
% gradient_y=gradient_y+D1gradient_y;
% elseif t>40 && t<41.2
% gradient_x=gradient_x+D2gradient_x;
% gradient_y=gradient_y+D2gradient_y;
% else 
% gradient_x=gradient_x;
% gradient_y=gradient_y;    
% end

% gradient_x=Gradient(1,1);
% gradient_y=Gradient(1,2);
gradient_z=0;
Gradient_all=[gradient_x;gradient_y;gradient_z];



Li=0.2;
Bi=[0,cos(pi/6),-cos(pi/6);
    -1,sin(pi/6),sin(pi/6);
    Li,Li,Li;];

R1=[cos(xa3),-sin(xa3),0;
    sin(xa3),cos(xa3),0;
    0,0,1;];
R=0.02;

gx=R1*inv(Bi')*R;
A=Gradient_all'*gx;
% A=[A;-gx];
%H=[1];
%H=[1,0;0,1];
%H=[0,0,0;0,0,0;0,0,0];

 H1=[1,0,0;0,1,0;0,0,0];
 H=(1/2)*gx'*H1*gx;
b=[0];
% b=[0;5000;5000;5000];
Gain=50;
Gradient_final=Gain*Gradient_all;
F=[-2*gx'*H1'*Gradient_final];
%=[];
u1=0;u2=0;u3=0;
U=PVF_optimizer(H,b,A,F,distance,gradient_x,gradient_y);

u1=U(1,1);
u2=U(2,1);
u3=U(3,1);

== matlab function scenario1_TAC_5robots_plus/agent_0/STL_barrier  ==
  data: b output; b1 output; yita output; h output; t input; p1 input; p2 input
function [b,b1,yita,h] = fcn(t,p1,p2)
if t<20
    d1=0;
    d2=100;
elseif t>=20 && t<40
    d1=0;
    d2=100;
else
    d1=100;
    d2=0;  
end

obs1=50;
obs2=50;
if t<20
b=145*exp(-0.24*t)+5-sqrt( (p1-d1)^2 + (p2-d2)^2 );
yita=-145*exp(-0.24*t)+5;
h=10-sqrt( (p1-d1)^2 + (p2-d2)^2 );
elseif t>=20 && t<40
    b=90*exp(-0.208*(t-20))+5-sqrt( (p1-d1)^2 + (p2-d2)^2 );
   yita=-90*exp(-0.2295*(t-20))+5;
    h=10-sqrt( (p1-d1)^2 + (p2-d2)^2 );
else
   b=145*exp(-0.24*(t-40))+5-sqrt( (p1-d1)^2 + (p2-d2)^2 );
   yita=-145*exp(-0.24*(t-40))+5;
   h=10-sqrt( (p1-d1)^2 + (p2-d2)^2 );
end
% b11=sqrt( (p1-x1_agent2)^2 + (p2-x2_agent2)^2 )-10 %collision avoidence with agent2
b12=sqrt( (p1-obs1)^2 + (p2-obs2)^2 )-20;%collision avoidence with obstacle (50,50)
% b13=sqrt( (p1-centerjk_1)^2 + (p2-centerjk_2)^2 )-R_jk_s;%collision avoidence with nominal
% b14=sqrt( (p1-60)^2 + (p2-85)^2 )-18; %static dynamic obstacle
% b15=sqrt( (p1-20)^2 + (p2-80)^2 )-10; %static dynamic obstacle


b1=-(1/20)*log(exp(-20*b12));

% b1=-(1/20)*log(exp(-20*b11)+exp(-20*b12)+exp(-20*b14)+exp(-20*b15));%+log(2);

== matlab function scenario1_TAC_5robots_plus/agent_1/STL_barrier  ==
  data: b output; b1 output; yita output; h output; t input; p1 input; p2 input; agent2_x1 input; agent2_x2 input; agent3_x1 input; agent3_x2 input; agent4_x1 input; agent4_x2 input; agent5_x1 input; agent5_x2 input; yita_1 output; h_1 output
function [b,b1,yita,h,yita_1,h_1] = fcn(t,p1,p2,agent2_x1,agent2_x2,agent3_x1,agent3_x2,agent4_x1,agent4_x2,agent5_x1,agent5_x2)
d11=0;d22=0;
if t<20
    d1=100;
    d2=100;
elseif t>=20 && t<41
    d1=0;d2=100;
    d11=0;d22=70;
else
    d1=100;
    d2=0;  
end

obs1=50;
obs2=50;
yita_1=0;h_1=0;
if t<20
% b=125*exp(-0.2295*t)+5-sqrt( (p1-d1)^2 + (p2-d2)^2 );
% yita=-125*exp(-0.2295*t)+5;
% h=10-sqrt( (p1-d1)^2 + (p2-d2)^2 );
b=145*exp(-0.24*t)+5-sqrt( (p1-d1)^2 + (p2-d2)^2 );
yita=-145*exp(-0.24*t)+5;
h=10-sqrt( (p1-d1)^2 + (p2-d2)^2 );
elseif t>=20 && t<41
    b_1=100*exp(-0.215*(t-20))+5-sqrt( (p1-d1)^2 + (p2-d2)^2 );
   yita_1=-100*exp(-0.215*(t-20))+5;
    h_1=10-sqrt( (p1-d1)^2 + (p2-d2)^2 );
    
   b_2=105*exp(-0.22*(t-20))+5-sqrt( (p1-d11)^2 + (p2-d22)^2 );
   yita=-105*exp(-0.22*(t-20))+5;
   h=10-sqrt( (p1-d11)^2 + (p2-d22)^2 );
   b=-(1/20)*log(exp(-20*b_1)+exp(-20*b_2));
else
   b=145*exp(-0.24*(t-40))+5-sqrt( (p1-d1)^2 + (p2-d2)^2 );
   yita=-145*exp(-0.24*(t-40))+5;
   h=10-sqrt( (p1-d1)^2 + (p2-d2)^2 );
end
% b11=sqrt( (p1-x1_agent2)^2 + (p2-x2_agent2)^2 )-10 %collision avoidence with agent2
bobs=sqrt( (p1-obs1)^2 + (p2-obs2)^2 )-20;%collision avoidence with obstacle (50,50)
b12=sqrt( (p1-agent2_x1)^2 + (p2-agent2_x2)^2 )-10;%collision avoidence with agent2
b13=sqrt( (p1-agent3_x1)^2 + (p2-agent3_x2)^2 )-10;%collision avoidence with agent3
b14=sqrt( (p1-agent4_x1)^2 + (p2-agent4_x2)^2 )-10;%collision avoidence with agent4
b15=sqrt( (p1-agent5_x1)^2 + (p2-agent5_x2)^2 )-10;%collision avoidence with agent5



b1=-(1/20)*log(exp(-20*bobs)+exp(-20*b12)+exp(-20*b13)+exp(-20*b14)+exp(-20*b15));

% b1=-(1/20)*log(exp(-20*b11)+exp(-20*b12)+exp(-20*b14)+exp(-20*b15));%+log(2);

== matlab function scenario1_TAC_5robots_plus/agent_1/MATLAB Function2 ==
  data: v1 input; v output; v2 input
function v = fcn(v1, v2)
v=sqrt(v1^2+v2^2);

== matlab function scenario1_TAC_5robots_plus/agent_1/velocity_constraint ==
  data: U1 input; Uc1 output; U2 input; U3 input; Uc2 output; Uc3 output; xa3 input; v_max input
function [Uc1,Uc2,Uc3] = fcn(U1,U2,U3,xa3,v_max)

Li=0.2;
Bi=[0,cos(pi/6),-cos(pi/6);
    -1,sin(pi/6),sin(pi/6);
    Li,Li,Li;];

R1=[cos(xa3),-sin(xa3),0;
    sin(xa3),cos(xa3),0;
    0,0,1;];
R=0.02;
gx=R1*inv(Bi')*R;

U=[U1;U2;U3];
V=[0;0;0];
V=gx*U;
if V(1,1)^2+V(2,1)^2<=v_max^2
     U(1,1)= U(1,1);
     U(2,1)= U(2,1);
else 
    U(1,1)=sqrt(v_max^2/(V(1,1)^2+V(2,1)^2))*U(1,1);
    U(2,1)=sqrt(v_max^2/(V(1,1)^2+V(2,1)^2))*U(2,1);
    U(3,1)=sqrt(v_max^2/(V(1,1)^2+V(2,1)^2))*U(3,1);
end

Uc1=U(1,1);
Uc2=U(2,1);
Uc3=U(3,1);

== matlab function scenario1_TAC_5robots_plus/agent_0/STL_controller ==
  data: x1 input; x2 input; b_in input; u1 output; xa3 input; u2 output; u3 output; t input; v_max input
function [u1,u2,u3]= fcn(x1, x2, b_in, xa3,t, v_max)
coder.extrinsic('quadoptimizer');
%coder.extrinsic('save');
if t<20
    d1=0; d2=100;
elseif t>=20 && t<40
   d1=0; d2=100; 
else
   d1=100; d2=0; 
end

partial_b=(1/2)*((x1-d1)^2+(x2-d2)^2)^(-1/2);
partial_b_x=[-2*partial_b*(x1-d1),-2*partial_b*(x2-d2),0];


Li=0.2;
Bi=[0,cos(pi/6),-cos(pi/6);
    -1,sin(pi/6),sin(pi/6);
    Li,Li,Li;];

R1=[cos(xa3),-sin(xa3),0;
    sin(xa3),cos(xa3),0;
    0,0,1;];
R=0.02;
gx=R1*inv(Bi')*R;

A=partial_b_x*gx;
% A=[A;-gx];
H=[1,0,0;0,1,0;0,0,1];
%H=[1];
if t<20
    b=20*b_in-0.24*145*exp(-0.24*t)-100;
elseif t>=20 && t<40
    b=20*b_in-0.208*90*exp(-0.208*(t-20))-100;
else
    b=20*b_in-0.24*145*exp(-0.24*(t-40))-100;
end
% b=[b;5000;5000;5000];


u1=0;u2=0;u3=0;
U=[0;0;0];
U=quadoptimizer(H,b,A);

%U=quadprod(H,[],-A,b);
% V=[0;0;0];
% V=gx*U;
% if V(1,1)^2+V(2,1)^2<=v_max^2
%      U(1,1)= U(1,1);
%      U(2,1)= U(2,1);
% else 
%     U(1,1)=sqrt(v_max^2/(V(1,1)^2+V(2,1)^2))*U(1,1);
%     U(2,1)=sqrt(v_max^2/(V(1,1)^2+V(2,1)^2))*U(2,1);
% end


u1=U(1,1);
u2=U(2,1);
u3=U(3,1);

== matlab function scenario1_TAC_5robots_plus/agent_0/omnidirectional robot_1 ==
  data: ua1 input; xa1_dot output; ua2 input; ua3 input; xa3 input; xa2_dot output; xa3_dot output
function [xa1_dot,xa2_dot,xa3_dot]= fcn(ua1,ua2,ua3,xa3)

Li=0.2;
Bi=[0,cos(pi/6),-cos(pi/6);
    -1,sin(pi/6),sin(pi/6);
    Li,Li,Li;];

R1=[cos(xa3),-sin(xa3),0;
    sin(xa3),cos(xa3),0;
    0,0,1;];
R=0.02;
A=R1*inv(Bi')*R*[ua1;ua2;ua3];
xa1_dot=A(1,1);
xa2_dot=A(2,1);
xa3_dot=A(3,1);

== matlab function scenario1_TAC_5robots_plus/agent_0/velocity_constraint ==
  data: U1 input; Uc1 output; U2 input; U3 input; Uc2 output; Uc3 output; xa3 input; v_max input
function [Uc1,Uc2,Uc3] = fcn(U1,U2,U3,xa3,v_max)

Li=0.2;
Bi=[0,cos(pi/6),-cos(pi/6);
    -1,sin(pi/6),sin(pi/6);
    Li,Li,Li;];

R1=[cos(xa3),-sin(xa3),0;
    sin(xa3),cos(xa3),0;
    0,0,1;];
R=0.02;
gx=R1*inv(Bi')*R;

U=[U1;U2;U3];
V=[0;0;0];
V=gx*U;
if V(1,1)^2+V(2,1)^2<=v_max^2
     U(1,1)= U(1,1);
     U(2,1)= U(2,1);
else 
    U(1,1)=sqrt(v_max^2/(V(1,1)^2+V(2,1)^2))*U(1,1);
    U(2,1)=sqrt(v_max^2/(V(1,1)^2+V(2,1)^2))*U(2,1);
    U(3,1)=sqrt(v_max^2/(V(1,1)^2+V(2,1)^2))*U(3,1);
end

Uc1=U(1,1);
Uc2=U(2,1);
Uc3=U(3,1);

== matlab function scenario1_TAC_5robots_plus/distance ==
  data: agent1_x1 input; distance_1_2 output; agent1_x2 input; agent2_x1 input; agent2_x2 input; agent3_x1 input; agent3_x2 input; agent4_x1 input; agent4_x2 input; agent5_x1 input; agent5_x2 input; distance_1_3 output; distance_1_4 output; distance_1_5 output; distance_2_3 output; distance_2_4 output; distance_2_5 output; distance_3_4 output; distance_3_5 output; distance_4_5 output
function [distance_1_2,distance_1_3,distance_1_4,distance_1_5,distance_2_3,distance_2_4,distance_2_5,distance_3_4,distance_3_5,distance_4_5]  = fcn(agent1_x1,agent1_x2,agent2_x1,agent2_x2,agent3_x1,agent3_x2,agent4_x1,agent4_x2,agent5_x1,agent5_x2)
distance_1_2=sqrt( (agent1_x1-agent2_x1)^2+ (agent1_x2-agent2_x2 )^2  );
distance_1_3=sqrt( (agent1_x1-agent3_x1)^2+ (agent1_x2-agent3_x2 )^2  );
distance_1_4=sqrt( (agent1_x1-agent4_x1)^2+ (agent1_x2-agent4_x2 )^2  );
distance_1_5=sqrt( (agent1_x1-agent5_x1)^2+ (agent1_x2-agent5_x2 )^2  );
distance_2_3=sqrt( (agent2_x1-agent3_x1)^2+ (agent2_x2-agent3_x2 )^2  );
distance_2_4=sqrt( (agent2_x1-agent4_x1)^2+ (agent2_x2-agent4_x2 )^2  );
distance_2_5=sqrt( (agent2_x1-agent5_x1)^2+ (agent2_x2-agent5_x2 )^2  );
distance_3_4=sqrt( (agent3_x1-agent4_x1)^2+ (agent3_x2-agent4_x2 )^2  );
distance_3_5=sqrt( (agent3_x1-agent5_x1)^2+ (agent3_x2-agent5_x2 )^2  );
distance_4_5=sqrt( (agent4_x1-agent5_x1)^2+ (agent4_x2-agent5_x2 )^2  );

== matlab function scenario1_TAC_5robots_plus/agent_3/MATLAB Function ==
  data: x1 input; theta output; y1 input
function theta = fcn(x1, y1)
theta=atan2(y1,x1);

== matlab function scenario1_TAC_5robots_plus/agent_3/MATLAB Function1 ==
  data: STL_u1 input; U1 output; STL_u2 input; STL_u3 input; PFM_u1 input; PFM_u2 input; PFM_u3 input; b1 input; U2 output; U3 output
function [U1,U2,U3] = fcn(STL_u1,STL_u2,STL_u3,PFM_u1,PFM_u2,PFM_u3,b1)
U_goal=[STL_u1;STL_u2;STL_u3];
U_obs=[PFM_u1;PFM_u2;PFM_u3];
k=0.15;
lambda=1-exp(-k*max(b1,0));
U=lambda*U_goal+(1-lambda)*U_obs;
U1=0;U2=0;U3=0;
U1=U(1,1);
U2=U(2,1);
U3=U(3,1);

== matlab function scenario1_TAC_5robots_plus/agent_3/MATLAB Function2 ==
  data: v1 input; v output; v2 input
function v = fcn(v1, v2)
v=sqrt(v1^2+v2^2);

== matlab function scenario1_TAC_5robots_plus/agent_3/Potential_Field_controller ==
  data: x1 input; x2 input; u1 output; xa3 input; agent1_x1 input; agent1_x2 input; agent2_x1 input; agent2_x2 input; agent4_x1 input; agent4_x2 input; agent5_x1 input; agent5_x2 input; t input; u2 output; u3 output; v_max input; yita output
function [u1,u2,u3,yita] = fcn(x1, x2, xa3,agent1_x1,agent1_x2,agent2_x1,agent2_x2,agent4_x1,agent4_x2,agent5_x1,agent5_x2,t,v_max)
coder.extrinsic('Calculate_gradient');
coder.extrinsic('Calculate_gradient_V1');
coder.extrinsic('Calculate_gradient_V1_yita');
coder.extrinsic('Calculate_gradient_static_d_1');
coder.extrinsic('Calculate_gradient_static_d_2');
coder.extrinsic('Calculate_gradient_dynamic');
coder.extrinsic('compute_convex_hull');
coder.extrinsic('PVF_optimizer');
coder.extrinsic('add_random');
yita=0;

A1=[-1,0;0,-1];
if t<20
    F=[100,0];
elseif t>=20 && t<41
     F=[200,200];
else
    F=[200,0];
end
obs=[50,50];
Robs_s=20;
r_obs=16;
distance=sqrt((x1-90)^2+(x2-90)^2);
gradient_x=0;gradient_y=0;
Dgradient_x=0;Dgradient_y=0;
agent1_gradient_x=0;agent1_gradient_y=0;
agent2_gradient_x=0;agent2_gradient_y=0;
agent4_gradient_x=0;agent4_gradient_y=0;
agent5_gradient_x=0;agent5_gradient_y=0;
[gradient_x,gradient_y]=Calculate_gradient(x1,x2,A1,F,50,50,Robs_s);
[agent1_gradient_x,agent1_gradient_y]=Calculate_gradient_dynamic(x1,x2,A1,F,agent1_x1,agent1_x2,10);
[agent2_gradient_x,agent2_gradient_y]=Calculate_gradient_dynamic(x1,x2,A1,F,agent2_x1,agent2_x2,10);
[agent4_gradient_x,agent4_gradient_y]=Calculate_gradient_dynamic(x1,x2,A1,F,agent4_x1,agent4_x2,10);
[agent5_gradient_x,agent5_gradient_y]=Calculate_gradient_dynamic(x1,x2,A1,F,agent5_x1,agent5_x2,10);
if sqrt((x1-agent1_x1)^2+(x2-agent1_x2)^2)<=30 %agent3 and agent1
     gradient_x=gradient_x+agent1_gradient_x;
     gradient_y=gradient_y+agent1_gradient_y;
end
if sqrt((x1-agent2_x1)^2+(x2-agent2_x2)^2)<=30 %agent3 and agent2
     gradient_x=gradient_x+agent2_gradient_x;
     gradient_y=gradient_y+agent2_gradient_y;
end
if sqrt((x1-agent4_x1)^2+(x2-agent4_x2)^2)<=30 %agent3 and agent4
     gradient_x=gradient_x+agent4_gradient_x;
     gradient_y=gradient_y+agent4_gradient_y;
end
if sqrt((x1-agent5_x1)^2+(x2-agent5_x2)^2)<=30 %agent3 and agent5
     gradient_x=gradient_x+agent5_gradient_x;
     gradient_y=gradient_y+agent5_gradient_y;
end
gradient_x=gradient_x;
gradient_y=gradient_y;  
gradient_z=0;
Gradient_all=[gradient_x;gradient_y;gradient_z];



Li=0.2;
Bi=[0,cos(pi/6),-cos(pi/6);
    -1,sin(pi/6),sin(pi/6);
    Li,Li,Li;];

R1=[cos(xa3),-sin(xa3),0;
    sin(xa3),cos(xa3),0;
    0,0,1;];
R=0.02;

gx=R1*inv(Bi')*R;
A=Gradient_all'*gx;
% A=[A;-gx];
%H=[1];
%H=[1,0;0,1];
%H=[0,0,0;0,0,0;0,0,0];

 H1=[1,0,0;0,1,0;0,0,0];
 H=(1/2)*gx'*H1*gx;
b=[0];
% b=[0;5000;5000;5000];
Gain=50;
Gradient_final=Gain*Gradient_all;
F=[-2*gx'*H1'*Gradient_final];
%=[];
u1=0;u2=0;u3=0;
U=PVF_optimizer(H,b,A,F,distance,gradient_x,gradient_y);

u1=U(1,1);
u2=U(2,1);
u3=U(3,1);

== matlab function scenario1_TAC_5robots_plus/agent_3/STL_barrier  ==
  data: b output; b1 output; yita output; h output; t input; p1 input; p2 input; agent1_x1 input; agent1_x2 input; agent2_x1 input; agent2_x2 input; agent4_x1 input; agent4_x2 input; agent5_x1 input; agent5_x2 input
function [b,b1,yita,h] = fcn(t,p1,p2,agent1_x1,agent1_x2,agent2_x1,agent2_x2,agent4_x1,agent4_x2,agent5_x1,agent5_x2)
if t<20
    d1=50;
    d2=0;
elseif t>=20 && t<41
    d1=100;
    d2=100;
else
    d1=100;
    d2=0;  
end

obs1=50;
obs2=50;
if t<20
b=105*exp(-0.22*t)+5-sqrt( (p1-d1)^2 + (p2-d2)^2 );
yita=-105*exp(-0.22*t)+5;
h=10-sqrt( (p1-d1)^2 + (p2-d2)^2 );
elseif t>=20 && t<41
    b=110*exp(-0.22*(t-20))+5-sqrt( (p1-d1)^2 + (p2-d2)^2 );
   yita=-110*exp(-0.22*(t-20))+5;
    h=10-sqrt( (p1-d1)^2 + (p2-d2)^2 );
else
   b=145*exp(-0.24*(t-40))+5-sqrt( (p1-d1)^2 + (p2-d2)^2 );
   yita=-145*exp(-0.24*(t-40))+5;
   h=10-sqrt( (p1-d1)^2 + (p2-d2)^2 );
end
% b11=sqrt( (p1-x1_agent2)^2 + (p2-x2_agent2)^2 )-10 %collision avoidence with agent2
bobs=sqrt( (p1-obs1)^2 + (p2-obs2)^2 )-20;%collision avoidence with obstacle (50,50)
b31=sqrt( (p1-agent1_x1)^2 + (p2-agent1_x2)^2 )-10;%collision avoidence with agent1
b32=sqrt( (p1-agent2_x1)^2 + (p2-agent2_x2)^2 )-10;%collision avoidence with agent2
b34=sqrt( (p1-agent4_x1)^2 + (p2-agent4_x2)^2 )-10;%collision avoidence with agent4
b35=sqrt( (p1-agent5_x1)^2 + (p2-agent5_x2)^2 )-10;%collision avoidence with agent5
% b13=sqrt( (p1-centerjk_1)^2 + (p2-centerjk_2)^2 )-R_jk_s;%collision avoidence with nominal
% b14=sqrt( (p1-60)^2 + (p2-85)^2 )-18; %static dynamic obstacle
% b15=sqrt( (p1-20)^2 + (p2-80)^2 )-10; %static dynamic obstacle


b1=-(1/20)*log(exp(-20*bobs)+exp(-20*b31)+exp(-20*b32)+exp(-20*b34)+exp(-20*b35));

% b1=-(1/20)*log(exp(-20*b11)+exp(-20*b12)+exp(-20*b14)+exp(-20*b15));%+log(2);
